simulink model "sampled_data_bilat_teleop_time_delay"  (R2017a)
settings: Solver=FixedStepAuto  StartTime=0.0  StopTime=10  FixedStep=0.0001  RelTol=1e-3
values from neighbouring files (symbols this model uses):
  Be = [0 0; 0 0]    [bilat_teleop_multiDOF_params.m]    (also in sampled_data_bilat_teleop_tavakoli_params.m = 0; sampled_data_bilat_teleop_time_delay_params.m = 0)
  Bh = [0 0; 0 0]    [bilat_teleop_multiDOF_params.m]    (also in sampled_data_bilat_teleop_tavakoli_params.m = 0.1; sampled_data_bilat_teleop_time_delay_params.m = 0.1)
  Bm = [1 0; 0 1]    [bilat_teleop_multiDOF_params.m]    (also in bilat_teleop_time_delay_params.m = 0; sampled_data_bilat_teleop_tavakoli_params.m = 0.1; sampled_data_bilat_teleop_time_delay_params.m = 0.1)
  Bs = [1 0; 0 1]    [bilat_teleop_multiDOF_params.m]    (also in bilat_teleop_time_delay_params.m = 0; sampled_data_bilat_teleop_tavakoli_params.m = 0.1; sampled_data_bilat_teleop_time_delay_params.m = 0.1)
  Kd = 1000    [Oct12workspace.mat]    (also in Test_apparatus_simulation.m = dd; bilat_teleop_time_delay_params.m = 0; custom_sim.m = 35; ode45_sim.m = 0)
  Ke = 0.142826110455    [Oct12workspace.mat]    (also in Test_apparatus_simulation.m; bilat_teleop_multiDOF_params.m = [0 0; 0 0]; sampled_data_bilat_teleop_tavakoli_params.m = 0; sampled_data_bilat_teleop_time_delay_params.m = 0)
  Kh = [0 0; 0 0]    [bilat_teleop_multiDOF_params.m]    (also in sampled_data_bilat_teleop_tavakoli_params.m = 0; sampled_data_bilat_teleop_time_delay_params.m = 0)
  Ki = 0    [bilat_teleop_time_delay_params.m]    (also in sampled_data_bilat_teleop_time_delay_params.m)
  Kp = 10000    [Oct12workspace.mat]    (also in Test_apparatus_simulation.m = pp; bilat_teleop_time_delay_params.m = 0; custom_sim.m = 100; ode45_sim.m = 100)
  Me = [0 0; 0 0]    [bilat_teleop_multiDOF_params.m]    (also in sampled_data_bilat_teleop_tavakoli_params.m = 0; sampled_data_bilat_teleop_time_delay_params.m = 0)
  Mh = [0 0; 0 0]    [bilat_teleop_multiDOF_params.m]    (also in sampled_data_bilat_teleop_tavakoli_params.m = 0.1; sampled_data_bilat_teleop_time_delay_params.m = 0.1)
  Mm = 1    [bilat_teleop_time_delay_params.m]    (also in sampled_data_bilat_teleop_tavakoli_params.m = 0.015; sampled_data_bilat_teleop_time_delay_params.m = 0.015)
  Ms = 1    [bilat_teleop_time_delay_params.m]    (also in sampled_data_bilat_teleop_tavakoli_params.m = 0.015; sampled_data_bilat_teleop_time_delay_params.m = 0.015)
  T1 = 0.001    [sampled_data_bilat_teleop_time_delay_params.m]
  T2 = 0.001    [sampled_data_bilat_teleop_time_delay_params.m]
  tsamp = 0.05    [sampled_data_bilat_teleop_tavakoli_params.m]    (also in sampled_data_bilat_teleop_time_delay_params.m = 0.005)
  xve = 0    [sampled_data_bilat_teleop_tavakoli_params.m]    (also in sampled_data_bilat_teleop_time_delay_params.m)
  xvh = 0    [sampled_data_bilat_teleop_tavakoli_params.m]    (also in sampled_data_bilat_teleop_time_delay_params.m)
libraries: simulink x2, dspstat3 x2
settings Model: Creator=salou  LastModifiedBy=salou
settings SolverCC: AutoInsertRateTranBlk=on  InsertRTBMode=Always

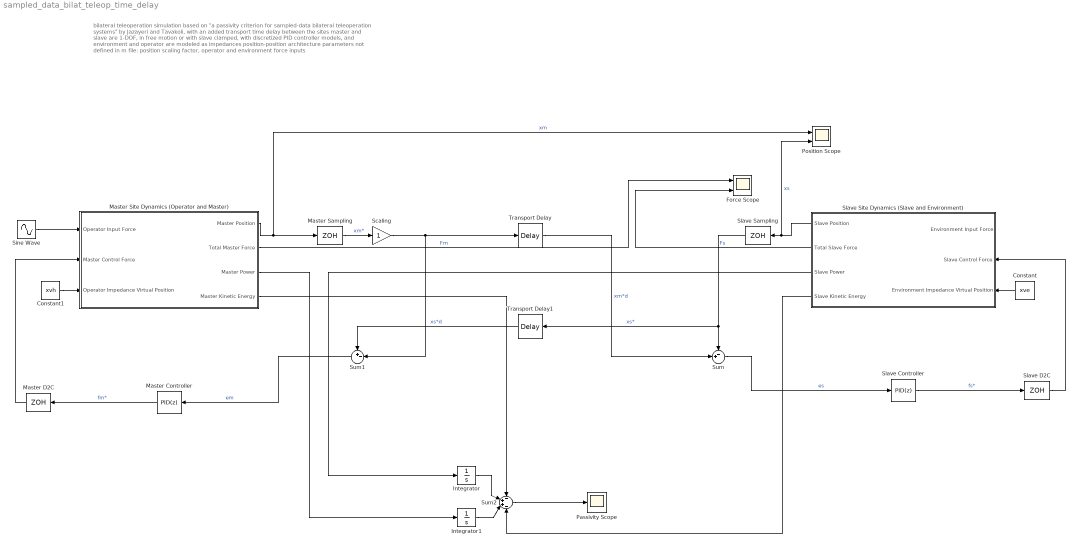
== system sampled_data_bilat_teleop_time_delay ==
  note: bilateral teleoperation simulation based on "a passivity criterion for sampled-data bilateral teleoperation systems" by Jazayeri and Tavakoli, with an added transport time delay between the sites
      |
      | master and slave are 1-DOF, in free motion or with slave clamped, with discretized PID controller models, and environment and operator are modeled as impedances
      |
      | position-position architecture
      |
      | parameters not defined in m file: position scaling factor, operator and environment force inputs
  Constant : Constant  Value=xve
  Constant1 : Constant  Value=xvh
  Force Scope : Scope  NumInputPorts=2
  Integrator : Integrator
  Integrator1 : Integrator
  Master Controller : simulink/Continuous/PID Controller  Controller=PID  TimeDomain=Discrete-time  SampleTime=-1  IntegratorMethod=Forward Euler  FilterMethod=Forward Euler  Form=Parallel  UseFilter=off  ControllerParametersSource=internal  P=Kp  I=Ki  D=Kd  N=100  InitialConditionSource=internal  InitialConditionForIntegrator=0  InitialConditionForFilter=0  ExternalReset=none  LimitOutput=off  UpperSaturationLimit=inf  LowerSaturationLimit=-inf  LinearizeAsGain=off  AntiWindupMode=none  Kb=1  TrackingMode=off  Kt=1  PParamMin=[]  PParamMax=[]  IParamMin=[]  IParamMax=[]  DParamMin=[]  DParamMax=[]  NParamMin=[]  NParamMax=[]  KbParamMin=[]  KbParamMax=[]  KtParamMin=[]  KtParamMax=[]  POutMin=[]  POutMax=[]  IOutMin=[]  IOutMax=[]  DOutMin=[]  DOutMax=[]  NOutMin=[]  NOutMax=[]  KbOutMin=[]  KbOutMax=[]  KtOutMin=[]  KtOutMax=[]  IntegratorOutMin=[]  IntegratorOutMax=[]  FilterOutMin=[]  FilterOutMax=[]  SumOutMin=[]  SumOutMax=[]  SumI1OutMin=[]  SumI1OutMax=[]  SumI2OutMin=[]  SumI2OutMax=[]  SumI3OutMin=[]  SumI3OutMax=[]  SumDOutMin=[]  SumDOutMax=[]  SaturationOutMin=[]  SaturationOutMax=[]  IntegratorContinuousStateAttributes=''  IntegratorStateMustResolveToSignalObject=off  IntegratorRTWStateStorageClass=Auto  FilterContinuousStateAttributes=''  FilterStateMustResolveToSignalObject=off  FilterRTWStateStorageClass=Auto  DifferentiatorICPrevScaledInput=0  DifferentiatorOutMin=[]  DifferentiatorOutMax=[]  InitialConditionSetting=State (most efficient)
  Master D2C : ZeroOrderHold  SampleTime=-1
  Master Sampling : ZeroOrderHold  SampleTime=tsamp
  Master Site Dynamics (Operator and Master) : Subsystem
  Passivity Scope : Scope
  Position Scope : Scope  NumInputPorts=2
  Scaling : Gain
  Sine Wave : Sin  Frequency=10  SampleTime=0
  Slave Controller : simulink/Continuous/PID Controller  Controller=PID  TimeDomain=Discrete-time  SampleTime=-1  IntegratorMethod=Forward Euler  FilterMethod=Forward Euler  Form=Parallel  UseFilter=off  ControllerParametersSource=internal  P=Kp  I=Ki  D=Kd  N=100  InitialConditionSource=internal  InitialConditionForIntegrator=0  InitialConditionForFilter=0  ExternalReset=none  LimitOutput=off  UpperSaturationLimit=inf  LowerSaturationLimit=-inf  LinearizeAsGain=off  AntiWindupMode=none  Kb=1  TrackingMode=off  Kt=1  PParamMin=[]  PParamMax=[]  IParamMin=[]  IParamMax=[]  DParamMin=[]  DParamMax=[]  NParamMin=[]  NParamMax=[]  KbParamMin=[]  KbParamMax=[]  KtParamMin=[]  KtParamMax=[]  POutMin=[]  POutMax=[]  IOutMin=[]  IOutMax=[]  DOutMin=[]  DOutMax=[]  NOutMin=[]  NOutMax=[]  KbOutMin=[]  KbOutMax=[]  KtOutMin=[]  KtOutMax=[]  IntegratorOutMin=[]  IntegratorOutMax=[]  FilterOutMin=[]  FilterOutMax=[]  SumOutMin=[]  SumOutMax=[]  SumI1OutMin=[]  SumI1OutMax=[]  SumI2OutMin=[]  SumI2OutMax=[]  SumI3OutMin=[]  SumI3OutMax=[]  SumDOutMin=[]  SumDOutMax=[]  SaturationOutMin=[]  SaturationOutMax=[]  IntegratorContinuousStateAttributes=''  IntegratorStateMustResolveToSignalObject=off  IntegratorRTWStateStorageClass=Auto  FilterContinuousStateAttributes=''  FilterStateMustResolveToSignalObject=off  FilterRTWStateStorageClass=Auto  DifferentiatorICPrevScaledInput=0  DifferentiatorOutMin=[]  DifferentiatorOutMax=[]  InitialConditionSetting=State (most efficient)
  Slave D2C : ZeroOrderHold  SampleTime=-1
  Slave Sampling : ZeroOrderHold  SampleTime=tsamp
  Slave Site Dynamics (Slave and Environment) : Subsystem
  Sum : Sum  Inputs=-+|
  Sum1 : Sum  Inputs=+-|
  Sum2 : Sum  Inputs=-++-
  Transport Delay : TransportDelay  DelayTime=T1
  Transport Delay1 : TransportDelay  DelayTime=T2
  wires:
  Master Site Dynamics (Operator and Master)/1(Master Position) -> Position Scope/1, Master Sampling/1  "xm"
  Slave Site Dynamics (Slave and Environment)/1(Slave Position) -> Position Scope/2, Slave Sampling/1  "xs"
  Master Sampling/1 -> Scaling/1  "xm*"
  Scaling/1 -> Sum1/2, Transport Delay/1
  Slave Sampling/1 -> Sum/1, Transport Delay1/1  "xs*"
  Sum/1 -> Slave Controller/1  "es"
  Master Controller/1 -> Master D2C/1  "fm*"
  Slave Controller/1 -> Slave D2C/1  "fs*"
  Master D2C/1 -> Master Site Dynamics (Operator and Master)/2(Master Control Force)
  Slave D2C/1 -> Slave Site Dynamics (Slave and Environment)/2(Slave Control Force)
  Sine Wave/1 -> Master Site Dynamics (Operator and Master)/1(Operator Input Force)
  Master Site Dynamics (Operator and Master)/2(Total Master Force) -> Force Scope/1  "Fm"
  Slave Site Dynamics (Slave and Environment)/2(Total Slave Force) -> Force Scope/2  "Fs"
  Master Site Dynamics (Operator and Master)/3(Master Power) -> Integrator1/1
  Slave Site Dynamics (Slave and Environment)/3(Slave Power) -> Integrator/1
  Integrator/1 -> Sum2/2
  Integrator1/1 -> Sum2/3
  Sum2/1 -> Passivity Scope/1
  Constant/1 -> Slave Site Dynamics (Slave and Environment)/3(Environment Impedance Virtual Position)
  Constant1/1 -> Master Site Dynamics (Operator and Master)/3(Operator Impedance Virtual Position)
  Transport Delay/1 -> Sum/2  "xm*d"
  Sum1/1 -> Master Controller/1  "em"
  Transport Delay1/1 -> Sum1/1  "xs*d"
  Master Site Dynamics (Operator and Master)/4(Master Kinetic Energy) -> Sum2/1
  Slave Site Dynamics (Slave and Environment)/4(Slave Kinetic Energy) -> Sum2/4

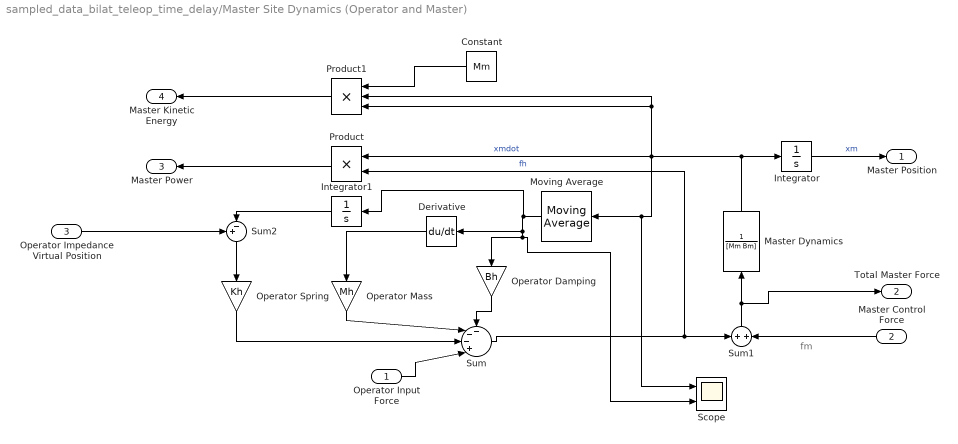
== system sampled_data_bilat_teleop_time_delay/Master Site Dynamics (Operator and Master) ==
  note: fm
  Operator Input Force : Inport
  Master Control Force : Inport  Port=2
  Operator Impedance Virtual Position : Inport  Port=3
  Constant : Constant  Value=Mm
  Derivative : Derivative
  Integrator : Integrator
  Integrator1 : Integrator
  Master Dynamics : TransferFcn  Denominator=[Mm Bm]
  Moving Average : dspstat3/Moving Average  Method=Sliding window  SpecifyWindowLength=on  WindowLength=150  ForgettingFactor=0.9  SimulateUsing=Code generation
  Operator Damping : Gain  Gain=Bh
  Operator Mass : Gain  Gain=Mh
  Operator Spring : Gain  Gain=Kh
  Product : Product
  Product1 : Product  Inputs=3
  Scope : Scope  NumInputPorts=2
  Sum : Sum  Inputs=---+|
  Sum1 : Sum  Inputs=+|+
  Sum2 : Sum  Inputs=+-|
  Master Position : Outport
  Total Master Force : Outport  Port=2
  Master Power : Outport  Port=3
  Master Kinetic Energy : Outport  Port=4
  wires:
  Operator Damping/1 -> Sum/1
  Sum1/1 -> Total Master Force/1, Master Dynamics/1
  Master Control Force/1 -> Sum1/2
  Operator Input Force/1 -> Sum/4
  Integrator/1 -> Master Position/1  "xm"
  Master Dynamics/1 -> Product1/2, Product1/3, Scope/1, Moving Average/1, Product/1, Integrator/1  "xmdot"
  Sum/1 -> Product/2, Sum1/1  "fh"
  Product/1 -> Master Power/1
  Operator Mass/1 -> Sum/2
  Moving Average/1 -> Integrator1/1, Derivative/1, Scope/2, Operator Damping/1
  Derivative/1 -> Operator Mass/1
  Integrator1/1 -> Sum2/2
  Operator Spring/1 -> Sum/3
  Operator Impedance Virtual Position/1 -> Sum2/1
  Sum2/1 -> Operator Spring/1
  Constant/1 -> Product1/1
  Product1/1 -> Master Kinetic Energy/1

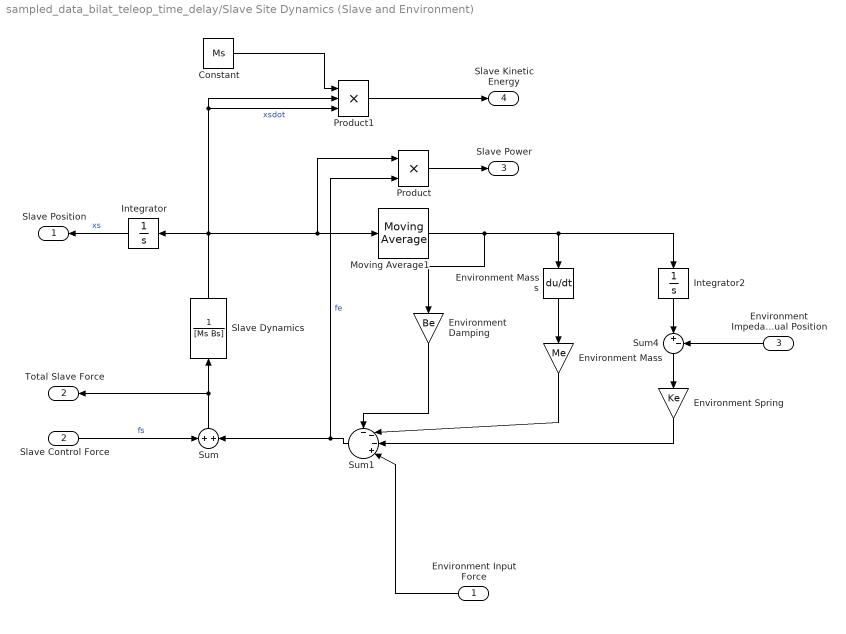
== system sampled_data_bilat_teleop_time_delay/Slave Site Dynamics (Slave and Environment) ==
  Environment Input Force : Inport
  Slave Control Force : Inport  Port=2
  Environment Impedance Virtual Position : Inport  Port=3
  Constant : Constant  Value=Ms
  Environment Damping : Gain  Gain=Be
  Environment Mass : Gain  Gain=Me
  Environment Mass s : Derivative
  Environment Spring : Gain  Gain=Ke
  Integrator : Integrator
  Integrator2 : Integrator
  Moving Average1 : dspstat3/Moving Average  Method=Sliding window  SpecifyWindowLength=on  WindowLength=150  ForgettingFactor=0.9  SimulateUsing=Code generation
  Product : Product
  Product1 : Product  Inputs=3
  Slave Dynamics : TransferFcn  Denominator=[Ms Bs]
  Sum : Sum  Inputs=+|+
  Sum1 : Sum  Inputs=---+|
  Sum4 : Sum  Inputs=|+-
  Slave Position : Outport
  Total Slave Force : Outport  Port=2
  Slave Power : Outport  Port=3
  Slave Kinetic Energy : Outport  Port=4
  wires:
  Integrator/1 -> Slave Position/1  "xs"
  Environment Input Force/1 -> Sum1/4
  Slave Control Force/1 -> Sum/1  "fs"
  Environment Damping/1 -> Sum1/1
  Slave Dynamics/1 -> Product1/3, Product1/2, Moving Average1/1, Product/1, Integrator/1  "xsdot"
  Sum1/1 -> Sum/2, Product/2  "fe"
  Sum/1 -> Slave Dynamics/1, Total Slave Force/1
  Environment Mass s/1 -> Environment Mass/1
  Product/1 -> Slave Power/1
  Moving Average1/1 -> Environment Damping/1, Integrator2/1, Environment Mass s/1
  Environment Mass/1 -> Sum1/2
  Integrator2/1 -> Sum4/1
  Environment Impedance Virtual Position/1 -> Sum4/2
  Sum4/1 -> Environment Spring/1
  Environment Spring/1 -> Sum1/3
  Constant/1 -> Product1/1
  Product1/1 -> Slave Kinetic Energy/1
